simulink model "mdlref_outdoor_temp"  (Simulink 6.0)
settings: Solver=ode3  SolverMode=SingleTasking  StartTime=0.0  StopTime=2*24*60*60  FixedStep=60  RelTol=1e-3  AbsTol=1e-6
settings Model: Creator=The MathWorks Inc.  LastModifiedBy=batserve  ExtModeAutoUpdateStatusClock=off
settings DataIOCC: ExternalInput=[]  InitialState=[]  LimitDataPoints=off  SaveOutput=off  SaveTime=off
settings OptimizationCC: BlockReduction=off  BooleanDataType=off  InlineParams=on
settings DebuggingCC: CheckExecutionContextPreStartOutputMsg=on  CheckExecutionContextRuntimeOutputMsg=on  SignalResolutionControl=UseLocalSettings  SolverPrmCheckMsg=none  IntegerOverflowMsg=none
settings HardwareCC: TargetUnknown=on

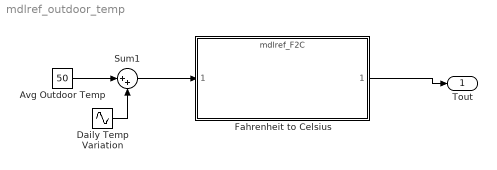
== system mdlref_outdoor_temp ==
  Avg Outdoor Temp : Constant  Value=50
  Daily Temp Variation : Sin  Amplitude=15  Frequency=2*pi/(24*3600)  SampleTime=0
  Fahrenheit to Celsius : ModelReference  ModelName=mdlref_F2C  ModelReferenceVersion=1.8  CopyOfModelName=mdlref_F2C
  Sum1 : Sum  Inputs=|++  SaturateOnIntegerOverflow=on  InputSameDT=on
  Tout : Outport
  wires:
  Fahrenheit to Celsius/1 -> Tout/1
  Avg Outdoor Temp/1 -> Sum1/1
  Sum1/1 -> Fahrenheit to Celsius/1
  Daily Temp Variation/1 -> Sum1/2
